simulink library "eps_model_lib"  (R2018b)
settings: Solver=VariableStepAuto  StartTime=0.0  StopTime=10.0  RelTol=1e-3
settings Model: Creator=Taylor  LastModifiedBy=Taylor

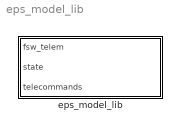
== system eps_model_lib ==
  eps_model_lib : Subsystem

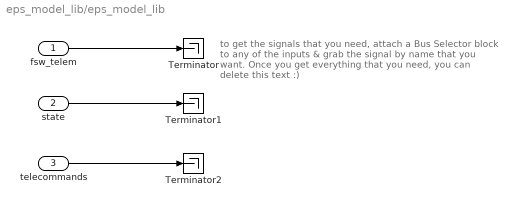
== system eps_model_lib/eps_model_lib ==
  note: to get the signals that you need, attach a
      | Bus Selector block to any of the inputs &
      | grab the signal by name that you want.
      |
      | Once you get everything that you need, you
      | can delete this text :)
  fsw_telem : Inport  OutDataTypeStr=Bus: fsw_telemetry
  state : Inport  Port=2  OutDataTypeStr=Bus: state
  telecommands : Inport  Port=3  OutDataTypeStr=Bus: cdh_data
  Terminator : Terminator
  Terminator1 : Terminator
  Terminator2 : Terminator
  wires:
  fsw_telem/1 -> Terminator/1
  state/1 -> Terminator1/1
  telecommands/1 -> Terminator2/1
